simulink model "FeedbackControl_SDV_harness"  (R2026a)
settings: Solver=FixedStepDiscrete  StartTime=0  StopTime=0.79000000000000004  FixedStep=0.01
PostLoadFcn:
  | Sldv.HarnessUtils.openMultiSimulationDesignStudy;
libraries: SignalEditorBlockLib x1, simulink x1
settings Model: DataDictionary=QuadData.sldd  SldvGeneratedHarnessModel=TestUnitModel=FeedbackControl|  Creator=The MathWorks, Inc.  LastModifiedBy=aylin.edgu
settings DataIOCC: ExternalInput=ds_faultB
settings OptimizationCC: ExpressionFolding=off
settings DebuggingCC: InheritedTsInSrcMsg=none
settings ModelReferenceCC: ModelReferenceNumInstancesAllowed=Single
settings RTWCC: SystemTargetFile=ert.tlc  GenerateMakefile=off  Description=Embedded Coder
settings ERTTargetCC: GenerateSampleERTMain=on
settings ConfigComp: CovEnable=on  CovScope=ReferencedModels  CovIncludeTopModel=off  CovMetricSettings=dcmoe  CovHTMLOptions=-aTS=1 -bRG=1 -bTC=0 -hTR=0 -nFC=0 -scm=1 -bcm=1  CovModelRefEnable=on

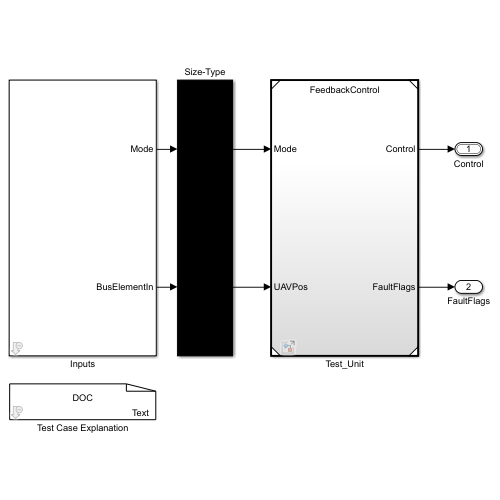
[thumbnail: Simulink's stored preview of the top-level diagram]
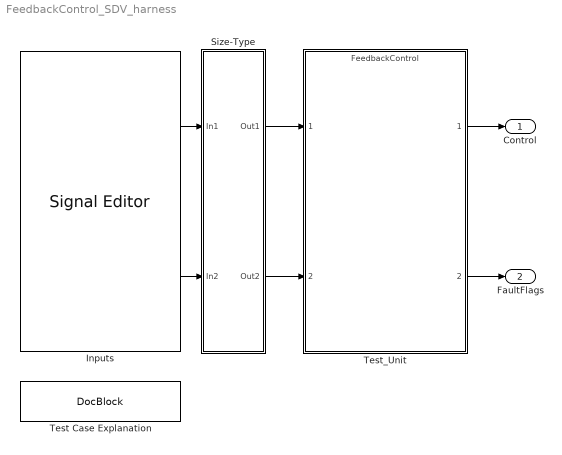
== system FeedbackControl_SDV_harness ==
  Inputs : SignalEditorBlockLib/Signal Editor  Tag=SignalEditorBlock  FileName=C:\UAV\VerificationBasedMBSE\FeedbackControl_harness_HarnessInputs.mat  ActiveScenario=TestCase_1  ActiveSignal=BusElementIn  IsBus=on  OutputBusObjectStr=Bus: MultirotorGuidanceStateBus  SampleTime=-1  Interpolate=off  ZeroCross=off  OutputAfterFinalValue=Setting to zero  Unit=inherit  PreserveSignalName=off  ApplySigPropsToAllScenarios=on  ApplySigPropsToAllSignals=off  SignalPropertySource=Dialog parameters
  Size-Type : Subsystem
  Test Case Explanation : simulink/Model-Wide Utilities/DocBlock  DocumentType=Text
  Test_Unit : ModelReference  ModelNameDialog=FeedbackControl  SimulationMode=Normal  ModelReferenceVersion=8.7
  Control : Outport  RequirementInfo={} %GIDa_0879a243_a871_47ae_a361_cfc044df0580  OutDataTypeStr=Bus: MultirotorGuidanceControlBus
  FaultFlags : Outport  RequirementInfo={} %GIDa_ad1314ed_f000_47af_8686_1b93920bfac5  Port=2
  wires:
  Inputs/1 -> Size-Type/1(In1)
  Test_Unit/1 -> Control/1
  Inputs/2 -> Size-Type/2(In2)
  Size-Type/1(Out1) -> Test_Unit/1
  Size-Type/2(Out2) -> Test_Unit/2
  Test_Unit/2 -> FaultFlags/1

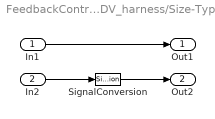
== system FeedbackControl_SDV_harness/Size-Type ==
  In1 : Inport
  In2 : Inport  Port=2
  SignalConversion : SignalConversion  ConversionOutput=Virtual bus  OverrideOpt=off
  Out1 : Outport
  Out2 : Outport  Port=2
  wires:
  In1/1 -> Out1/1
  In2/1 -> SignalConversion/1
  SignalConversion/1 -> Out2/1
